simulink model "SM_MotCD"  (R2023b)
settings: Solver=VariableStepAuto  StartTime=0.0  StopTime=10.0  RelTol=1e-3
values from neighbouring files (symbols this model uses):
  B = 0.0012    [MotCD.m]    (also in MotCD.mat)
  J = 0.001    [MotCD.m]    (also in MotCD.mat)
  K = 0.01    [MotCD.m]    (also in MotCD.mat)
  L = 0.023    [MotCD.m]    (also in MotCD.mat)
  R = 2    [MotCD.m]    (also in MotCD.mat)

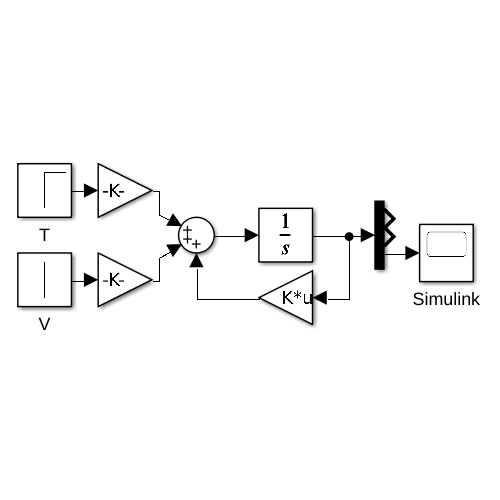
[thumbnail: Simulink's stored preview of the top-level diagram]
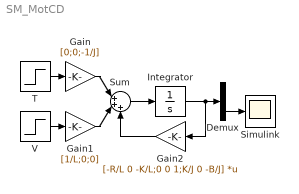
== system SM_MotCD ==
  Demux : Demux  Outputs=3
  Gain : Gain  Gain=[0;0;-1/J]
  Gain1 : Gain  Gain=[1/L;0;0]
  Gain2 : Gain  Gain=[-R/L 0 -K/L;0 0 1;K/J 0 -B/J]  Multiplication=Matrix(K*u)
  Integrator : Integrator
  Simulink : Scope
  Sum : Sum  Inputs=|+++
  T : Step  Time=0  After=0  SampleTime=0
  V : Step  Time=0  After=5  SampleTime=0
  wires:
  T/1 -> Gain/1
  V/1 -> Gain1/1
  Sum/1 -> Integrator/1
  Integrator/1 -> Gain2/1, Demux/1
  Gain2/1 -> Sum/3
  Gain1/1 -> Sum/2
  Gain/1 -> Sum/1
  Demux/3 -> Simulink/1
